simulink model "Citation_FlightGear_v2"  (R2026a)
settings: Solver=ode5  StopTime=40  FixedStep=0.01  EnableMultiTasking=on
InitFcn:
  | run('initcit.m')
  | run('id_init.m')
values from neighbouring files (symbols this model uses):
  cv1 = 20000    [gear_params.m]
  cv2 = cv1    (= 20000)    [gear_params.m]
  cv3 = 4000    [gear_params.m]
  cv4 = 20000    [gear_params.m]
  deltagmax1 = 0.25    [gear_params.m]
  deltagmax2 = deltagmax1    (= 0.25)    [gear_params.m]
  deltagmax3 = 0.24    [gear_params.m]
  deltagmax4 = 0.02    [gear_params.m]
  kt1 = 525020    [gear_params.m]
  kt2 = kt1    (= 525020)    [gear_params.m]
  kt3 = 457050    [gear_params.m]
  murol = 0.03*10    (= 0.3)    [gear_params.m]
  P1 = 2000    [gear_params.m]
  P2 = P1    (= 2000)    [gear_params.m]
  P3 = 2550    [gear_params.m]
  P4 = 40000    [gear_params.m]
  PL0 = 10000*eye(6)    [id_init.m]
  PM0 = 10000*eye(4)    [id_init.m]
  PN0 = 10000*eye(6)    [id_init.m]
  PX0 = 10000*eye(5)    [id_init.m]
  PY0 = 10000*eye(6)    [id_init.m]
  PZ0 = 10000*eye(4)    [id_init.m]
  thetaL0 = zeros(6,1)    [id_init.m]
  thetaM0 = zeros(4,1)    [id_init.m]
  thetaN0 = zeros(6,1)    [id_init.m]
  thetaX0 = zeros(5,1)    [id_init.m]
  thetaY0 = zeros(6,1)    [id_init.m]
  thetaZ0 = zeros(4,1)    [id_init.m]
  TL = 7.0875e-06    [id_init.m]    (also in plot_comparison_step_4.m = T_var(4))
  TM = 3.2564e-06    [id_init.m]    (also in plot_comparison_step_4.m = T_var(5))
  TN = 5.4692e-07    [id_init.m]    (also in plot_comparison_step_4.m = T_var(6))
  TX = 2.2784e-06    [id_init.m]    (also in plot_comparison_step_4.m = T_var(1))
  TY = 8.0633e-07    [id_init.m]    (also in plot_comparison_step_4.m = T_var(2))
  TZ = 2.8004e-05    [id_init.m]    (also in plot_comparison_step_4.m = T_var(3))
  xl1 = xcg-6.858    [gear_params.m]
  xl2 = xcg-6.858    [gear_params.m]
  xl3 = xcg-2.0752    [gear_params.m]
  xl4 = xcg-12.742    [gear_params.m]
  yl1 = 1.918    [gear_params.m]
  yl2 = -1.918    [gear_params.m]
  yl3 = 0    [gear_params.m]
  yl4 = 0    [gear_params.m]
  zl1 = zcg-1.701    [gear_params.m]
  zl2 = zcg-1.701    [gear_params.m]
  zl3 = zcg-1.7488    [gear_params.m]
  zl4 = zcg-2.78    [gear_params.m]
undefined symbols (not defined in the file or in its folder): chord, Deng, ealphag, ealphas, g0, hDME, hGS, lh, massinit, matbuaf, matdaf, matdam, matdbbf, matdeaf, matdgaf, matdqaf, matduaf, matdwaw, matedhr, mateif, matelhr, matemhr, matemv1, matemv2, matemve, matetam, mateuaf, matfaaf, matfaxl, matff, matibaf, matibb, matibmh, matipaf, matipmh, matiraf, matiuaf, matiwaf, matlaf, matlam, matleaf, matleam, matlgaf, matlqaf, matluaf, matmaaf, matmaam, matmaf, matmam, matmbbf, matmeaf, matmeam, matmgaf, matmqaf, matmrbr, matn1d, matn2d, matnbab, matnbaf, matnbmh ... (+53)
libraries: simulink x12, aerolibfltsims x3, aerolibconvert2 x2, aerolibobsolete x1, aerolibanimutils x1
(part 2 of 5)

== system Citation_FlightGear_v2/Cessna Citation 500/Citation model DASMAT/AIRCRAFT MODEL/EQM ==
  "FMtot " : Inport
  FMa : Inport  Port=2
  FMadot : Inport  Port=3
  FMbdot : Inport  Port=4
  massinit : Inport  Port=5
  wind : Inport  Port=6
  CFMa correction : Subsystem
  Integrator : Integrator  InitialCondition=x0
  State Derivatives : Subsystem
  x : Outport
  xdot : Outport  Port=2
  yuvw : Outport  Port=3
  FMtot corrected : Outport  Port=4
  FMa corrected : Outport  Port=5
  wires:
  State Derivatives/2(yuvw) -> yuvw/1
  State Derivatives/3(FMtot corrected) -> FMtot corrected/1
  FMa/1 -> CFMa correction/2(FMa)
  State Derivatives/1(xdot) -> xdot/1, CFMa correction/1(xdot), Integrator/1
  CFMa correction/1(FMa corrected) -> FMa corrected/1
  massinit/1 -> State Derivatives/5(massinit)
  "FMtot "/1 -> State Derivatives/2(FMtot)
  FMadot/1 -> CFMa correction/3(FMadot), State Derivatives/3(FMadot)
  FMbdot/1 -> CFMa correction/4(FMbdot), State Derivatives/4(FMbdot)
  Integrator/1 -> State Derivatives/1(x), x/1
  wind/1 -> State Derivatives/6(wind)

== system Citation_FlightGear_v2/Cessna Citation 500/Citation model DASMAT/AIRCRAFT MODEL/FM SORT ==
  FMa : Inport
  FMag : Inport  Port=2
  FMt : Inport  Port=3
  "Fgr " : Inport  Port=4
  Fgear : Inport  Port=5
  Mux : Mux  Inputs=[12 12]
  Sum : Sum  Inputs=+++++  InputSameDT=on  SaturateOnIntegerOverflow=on  OutDataTypeStr=Inherit: Same as first input
  Sum1 : Sum  Inputs=++++  InputSameDT=on  SaturateOnIntegerOverflow=on  OutDataTypeStr=Inherit: Same as first input
  aero : Demux  Outputs=[12 12]
      settings: DisplayOption=none
  engine : Demux  Outputs=[12 12]
      settings: DisplayOption=none
  gear : Demux  Outputs=[12 12]
      settings: DisplayOption=none
  gust : Demux  Outputs=[12 12]
      settings: DisplayOption=none
  FMtot : Outport
  wires:
  FMt/1 -> engine/1
  FMa/1 -> aero/1
  FMag/1 -> gust/1
  gust/2 -> Sum1/2
  Sum1/1 -> Mux/2
  engine/2 -> Sum1/3
  aero/2 -> Sum1/1
  gust/1 -> Sum/2
  engine/1 -> Sum/3
  Sum/1 -> Mux/1
  "Fgr "/1 -> Sum/4
  aero/1 -> Sum/1
  Mux/1 -> FMtot/1
  Fgear/1 -> gear/1
  gear/1 -> Sum/5
  gear/2 -> Sum1/4

== system Citation_FlightGear_v2/Cessna Citation 500/Citation model DASMAT/AIRCRAFT MODEL/GRAVITY ==
  "x " : Inport
  massinit : Inport  Port=2
  yatm : Inport  Port=3
  Fgr transformation : S-Function  FunctionName=ac_axes  Parameters=3  SFunctionDeploymentMode=off  EnableBusSupport=off
  Mux : Mux  Inputs=[12 3]
  Mux1 : Mux  Inputs=3
  Terminator_{1..9} (9 alike) : Terminator
  W : Product  InputSameDT=on  SaturateOnIntegerOverflow=on  OutDataTypeStr=Inherit: Same as first input
  atmosphere : Demux  Outputs=8
      settings: DisplayOption=none
  mass cg inertia : Demux  Outputs=[1 3 4]
      settings: DisplayOption=none
  zero : Constant  Value=0
  Fgr : Outport
  wires:
  mass cg inertia/3 -> Terminator_9/1
  mass cg inertia/2 -> Terminator_8/1
  atmosphere/8 -> Terminator_7/1
  atmosphere/7 -> Terminator_6/1
  atmosphere/6 -> Terminator_5/1
  atmosphere/5 -> Terminator_4/1
  atmosphere/3 -> Terminator_3/1
  atmosphere/2 -> Terminator_2/1
  atmosphere/1 -> Terminator_1/1
  Mux/1 -> Fgr transformation/1
  "x "/1 -> Mux/1
  Fgr transformation/1 -> Fgr/1
  mass cg inertia/1 -> W/1
  massinit/1 -> mass cg inertia/1
  yatm/1 -> atmosphere/1
  W/1 -> Mux1/3
  Mux1/1 -> Mux/2
  zero/1 -> Mux1/1, Mux1/2
  atmosphere/4 -> W/2

== system Citation_FlightGear_v2/Cessna Citation 500/Citation model DASMAT/AIRCRAFT MODEL/LANDING GEAR ==
  note: Landing Gear Model
      | Cessna Citation 500
      | Version 0.04NLR
      | (c) A.R. Veldhuijzen September 2001
  x : Inport
  xdot : Inport  Port=2
  massinit : Inport  Port=3
  ua : Inport  Port=4
  terr elev : Inport  Port=5
  Gear axes-cg transformation : Subsystem
  Landing Gear model : Subsystem
  Switch : Switch  Threshold=0.95  InputSameDT=off
  gear position : Selector  IndexOptions=Index vector (dialog)  Indices=[8]  OutputSizes=1
  zero : Constant  Value=[0 0 0 0 0 0]
  Fmt : Outport
  wires:
  xdot/1 -> Landing Gear model/2(xdot)
  x/1 -> Landing Gear model/1(x), Gear axes-cg transformation/2("x ")
  massinit/1 -> Gear axes-cg transformation/3(massinit)
  Gear axes-cg transformation/1(FMt) -> Fmt/1
  zero/1 -> Switch/1
  Landing Gear model/1(Forces and Moments) -> Switch/3
  Switch/1 -> Gear axes-cg transformation/1(FMt model)
  ua/1 -> gear position/1
  gear position/1 -> Switch/2
  terr elev/1 -> Landing Gear model/3(terrain elevation)

== system Citation_FlightGear_v2/Cessna Citation 500/Citation model DASMAT/AIRCRAFT MODEL/OBSERVATIONS ==
  note: Modified by Alex : Flight-Path Subsystem from Ac_mod instead of Ac_modpc
  x : Inport
  xdot : Inport  Port=2
  yuvw : Inport  Port=3
  FMtot : Inport  Port=4
  FMa : Inport  Port=5
  Fgr : Inport  Port=6
  massinit : Inport  Port=7
  yatm : Inport  Port=8
  Acceleration : Subsystem
  Energy : Subsystem
  Flight-Path : Subsystem
  yacc : Outport
  yfp : Outport  Port=2
  ys : Outport  Port=3
  wires:
  yuvw/1 -> Flight-Path/3(yuvw)
  Flight-Path/1(yfp) -> yfp/1
  Energy/1(ys) -> ys/1
  Acceleration/1(yacc) -> yacc/1
  FMa/1 -> Acceleration/4(FMa)
  Fgr/1 -> Acceleration/5(Fgr)
  yatm/1 -> Energy/3(yatm)
  FMtot/1 -> Acceleration/3(FMtot)
  Acceleration/2(acc earth) -> Flight-Path/4(acc earth)
  x/1 -> Flight-Path/1(x), Energy/1(x), Acceleration/1(x)
  xdot/1 -> Flight-Path/2(xdot), Energy/2(xdot), Acceleration/2(xdot)
  massinit/1 -> Acceleration/6(massinit)

== system Citation_FlightGear_v2/Cessna Citation 500/Citation model DASMAT/AIRCRAFT MODEL/WIND//TURBULENCE ==
  "x " : Inport
  Logarithmic Wind model : Subsystem
  Mux : Mux  Inputs=[12 3]
  Vwind transformation : S-Function  FunctionName=ac_axes  Parameters=3  SFunctionDeploymentMode=off  EnableBusSupport=off
  wind : Outport
  wires:
  Mux/1 -> Vwind transformation/1
  Vwind transformation/1 -> wind/1
  "x "/1 -> Mux/1, Logarithmic Wind model/1(In1)
  Logarithmic Wind model/1(Out1) -> Mux/2

== system Citation_FlightGear_v2/Pilot/Virtual Joystick (if you don't have a real one!)/Virtual Joystick/Throttle setting ==
  Demux : Demux  Tag=STV Demux  Outputs=1
      settings: DisplayOption=none
  FromWs : FromWorkspace  Tag=STV FromWs  VariableName=tuvar
      SigBuilderData=|
      | common.afterFinalStr = 'Extrapolate'
      | common.sampleTime = 0
      | dataSet.timeRange = [0 30]
      | dataSet.name = 'Group 1'
      | sbobj.Groups.Name = 'Group 1'
      | sbobj.Groups.Signals.Name = 'Signal 1'
      | sbobj.Groups.Signals.XData = [0 30]
      | sbobj.Groups.Signals.YData = [0.695 0.695]
      | sbobj.Groups.TimeRange = [0 30]
  Signal 1 : Outport  Tag=STV Outport
  wires:
  Demux/1 -> Signal 1/1
  FromWs/1 -> Demux/1

== system Citation_FlightGear_v2/Pilot/Virtual Joystick (if you don't have a real one!)/Virtual Joystick/delta aileron ==
  Demux : Demux  Tag=STV Demux  Outputs=3
      settings: DisplayOption=none
  FromWs : FromWorkspace  Tag=STV FromWs  VariableName=tuvar
      SigBuilderData=|
      | common.afterFinalStr = 'Extrapolate'
      | common.sampleTime = 0
      | dataSet.timeRange = [0 40]
      | dataSet.name = 'Group 1'
      | sbobj.Groups.Name = 'Group 1'
      | sbobj.Groups.Signals(1).Name = 'Signal 1'
      | sbobj.Groups.Signals(1).XData = [0 5 5 18 18 40]
      | sbobj.Groups.Signals(1).YData = [0 0 0.152 0.152 0 0]
      | sbobj.Groups.Signals(2).Name = 'Signal 2'
      | sbobj.Groups.Signals(2).XData = [0 25 25 28 28 40]
      | sbobj.Groups.Signals(2).YData = [0 0 -0.07 -0.07 0 0]
      | sbobj.Groups.Signals(3).Name = 'Signal 3'
      | sbobj.Groups.Signals(3).XData = [0 28 28 40]
      | sbobj.Groups.Signals(3).YData = [0 0 -0.04 -0.04]
      | sbobj.Groups.TimeRange = [0 40]
  Signal 1 : Outport  Tag=STV Outport
  Signal 2 : Outport  Tag=STV Outport  Port=2
  Signal 3 : Outport  Tag=STV Outport  Port=3
  wires:
  Demux/1 -> Signal 1/1
  FromWs/1 -> Demux/1
  Demux/2 -> Signal 2/1
  Demux/3 -> Signal 3/1

== system Citation_FlightGear_v2/Pilot/Virtual Joystick (if you don't have a real one!)/Virtual Joystick/delta elevator ==
  Demux : Demux  Tag=STV Demux  Outputs=1
      settings: DisplayOption=none
  FromWs : FromWorkspace  Tag=STV FromWs  VariableName=tuvar
      SigBuilderData=|
      | common.afterFinalStr = 'Extrapolate'
      | common.sampleTime = 0
      | dataSet.timeRange = [0 100]
      | dataSet.name = 'Group 1'
      | sbobj.Groups.Name = 'Group 1'
      | sbobj.Groups.Signals.Name = 'Signal 1'
      | sbobj.Groups.Signals.XData = [0 5 100]
      | sbobj.Groups.Signals.YData = [-0.02795 -0.02795 -0.02795]
      | sbobj.Groups.TimeRange = [0 100]
  Signal 1 : Outport  Tag=STV Outport
  wires:
  Demux/1 -> Signal 1/1
  FromWs/1 -> Demux/1

== system Citation_FlightGear_v2/Pilot/Virtual Joystick (if you don't have a real one!)/Virtual Joystick/delta rudder ==
  Demux : Demux  Tag=STV Demux  Outputs=1
      settings: DisplayOption=none
  FromWs : FromWorkspace  Tag=STV FromWs  VariableName=tuvar
      SigBuilderData=|
      | common.afterFinalStr = 'Extrapolate'
      | common.sampleTime = 0
      | dataSet.timeRange = [0 30]
      | dataSet.name = 'Group 1'
      | sbobj.Groups.Name = 'Group 1'
      | sbobj.Groups.Signals.Name = 'Signal 1'
      | sbobj.Groups.Signals.XData = [0 4 6 30]
      | sbobj.Groups.Signals.YData = [0 0 0 0]
      | sbobj.Groups.TimeRange = [0 30]
  Signal 1 : Outport  Tag=STV Outport
  wires:
  Demux/1 -> Signal 1/1
  FromWs/1 -> Demux/1

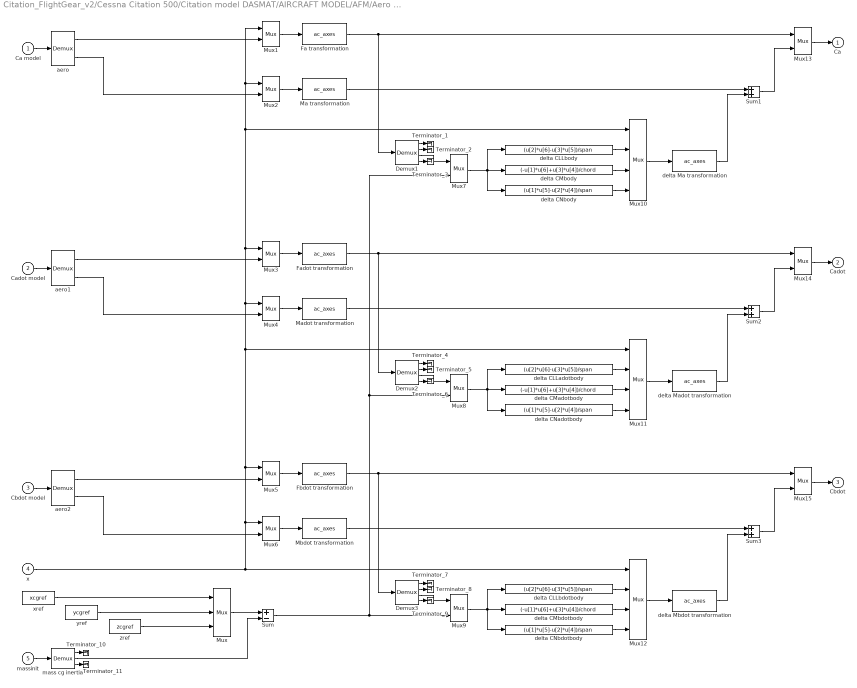
== system Citation_FlightGear_v2/Cessna Citation 500/Citation model DASMAT/AIRCRAFT MODEL/AFM/Aero axes-cg transformation ==
  Ca model : Inport
  Cadot model : Inport  Port=2
  Cbdot model : Inport  Port=3
  "x " : Inport  Port=4
  massinit : Inport  Port=5
  Demux1 : Demux  Outputs=[3 3 3 3]
      settings: DisplayOption=none
  Demux2 : Demux  Outputs=[3 3 3 3]
      settings: DisplayOption=none
  Demux3 : Demux  Outputs=[3 3 3 3]
      settings: DisplayOption=none
  Fa transformation : S-Function  FunctionName=ac_axes  Parameters=axes_CFMaero  SFunctionDeploymentMode=off  EnableBusSupport=off
  Fadot transformation : S-Function  FunctionName=ac_axes  Parameters=axes_CFMaero  SFunctionDeploymentMode=off  EnableBusSupport=off
  Fbdot transformation : S-Function  FunctionName=ac_axes  Parameters=axes_CFMaero  SFunctionDeploymentMode=off  EnableBusSupport=off
  Ma transformation : S-Function  FunctionName=ac_axes  Parameters=axes_CFMaero  SFunctionDeploymentMode=off  EnableBusSupport=off
  Madot transformation : S-Function  FunctionName=ac_axes  Parameters=axes_CFMaero  SFunctionDeploymentMode=off  EnableBusSupport=off
  Mbdot transformation : S-Function  FunctionName=ac_axes  Parameters=axes_CFMaero  SFunctionDeploymentMode=off  EnableBusSupport=off
  Mux : Mux  Inputs=3
  Mux{1..6} (6 alike) : Mux  Inputs=[12 3]
  Mux10 : Mux  Inputs=[12 1 1 1]
  Mux11 : Mux  Inputs=[12 1 1 1]
  Mux12 : Mux  Inputs=[12 1 1 1]
  Mux13 : Mux  Inputs=[12 12]
  Mux14 : Mux  Inputs=[12 12]
  Mux15 : Mux  Inputs=[12 12]
  Mux7 : Mux  Inputs=[3 3]
  Mux8 : Mux  Inputs=[3 3]
  Mux9 : Mux  Inputs=[3 3]
  Sum : Sum  Inputs=+-  InputSameDT=on  SaturateOnIntegerOverflow=on  OutDataTypeStr=Inherit: Same as first input
  Sum1 : Sum  InputSameDT=on  SaturateOnIntegerOverflow=on  OutDataTypeStr=Inherit: Same as first input
  Sum2 : Sum  InputSameDT=on  SaturateOnIntegerOverflow=on  OutDataTypeStr=Inherit: Same as first input
  Sum3 : Sum  InputSameDT=on  SaturateOnIntegerOverflow=on  OutDataTypeStr=Inherit: Same as first input
  Terminator_{1..11} (11 alike) : Terminator
  aero : Demux  Outputs=[3 3]
      settings: DisplayOption=none
  aero1 : Demux  Outputs=[3 3]
      settings: DisplayOption=none
  aero2 : Demux  Outputs=[3 3]
      settings: DisplayOption=none
  delta CLLadotbody : Fcn  Expr=(u[2]*u[6]-u[3]*u[5])/span
  delta CLLbdotbody : Fcn  Expr=(u[2]*u[6]-u[3]*u[5])/span
  delta CLLbody : Fcn  Expr=(u[2]*u[6]-u[3]*u[5])/span
  delta CMadotbody : Fcn  Expr=(-u[1]*u[6]+u[3]*u[4])/chord
  delta CMbdotbody : Fcn  Expr=(-u[1]*u[6]+u[3]*u[4])/chord
  delta CMbody : Fcn  Expr=(-u[1]*u[6]+u[3]*u[4])/chord
  delta CNadotbody : Fcn  Expr=(u[1]*u[5]-u[2]*u[4])/span
  delta CNbdotbody : Fcn  Expr=(u[1]*u[5]-u[2]*u[4])/span
  delta CNbody : Fcn  Expr=(u[1]*u[5]-u[2]*u[4])/span
  delta Ma transformation : S-Function  FunctionName=ac_axes  Parameters=2  SFunctionDeploymentMode=off  EnableBusSupport=off
  delta Madot transformation : S-Function  FunctionName=ac_axes  Parameters=2  SFunctionDeploymentMode=off  EnableBusSupport=off
  delta Mbdot transformation : S-Function  FunctionName=ac_axes  Parameters=2  SFunctionDeploymentMode=off  EnableBusSupport=off
  mass cg inertia : Demux  Outputs=[1 3 4]
      settings: DisplayOption=none
  xref : Constant  Value=xcgref
  yref : Constant  Value=ycgref
  zref : Constant  Value=zcgref
  Ca : Outport
  Cadot : Outport  Port=2
  Cbdot : Outport  Port=3
  wires:
  mass cg inertia/3 -> Terminator_11/1
  mass cg inertia/1 -> Terminator_10/1
  Demux3/4 -> Terminator_9/1
  Demux3/2 -> Terminator_8/1
  Demux3/1 -> Terminator_7/1
  Demux2/4 -> Terminator_6/1
  Demux2/2 -> Terminator_5/1
  Demux2/1 -> Terminator_4/1
  Demux1/4 -> Terminator_3/1
  Demux1/2 -> Terminator_2/1
  Demux1/1 -> Terminator_1/1
  aero1/1 -> Mux3/2
  Cadot model/1 -> aero1/1
  aero1/2 -> Mux4/2
  Ca model/1 -> aero/1
  massinit/1 -> mass cg inertia/1
  aero/1 -> Mux1/2
  xref/1 -> Mux/1
  yref/1 -> Mux/2
  zref/1 -> Mux/3
  mass cg inertia/2 -> Sum/2
  Mux/1 -> Sum/1
  Fa transformation/1 -> Demux1/1, Mux13/1
  Mux7/1 -> delta CLLbody/1, delta CNbody/1, delta CMbody/1
  delta CLLbody/1 -> Mux10/2
  delta CMbody/1 -> Mux10/3
  delta CNbody/1 -> Mux10/4
  Mux10/1 -> delta Ma transformation/1
  Ma transformation/1 -> Sum1/1
  Sum1/1 -> Mux13/2
  Mux13/1 -> Ca/1
  Mux1/1 -> Fa transformation/1
  Mux3/1 -> Fadot transformation/1
  Mux14/1 -> Cadot/1
  Sum2/1 -> Mux14/2
  Madot transformation/1 -> Sum2/1
  Mux12/1 -> delta Mbdot transformation/1
  delta CNbdotbody/1 -> Mux12/4
  delta CMbdotbody/1 -> Mux12/3
  delta CLLbdotbody/1 -> Mux12/2
  Mux9/1 -> delta CLLbdotbody/1, delta CNbdotbody/1, delta CMbdotbody/1
  Mux4/1 -> Madot transformation/1
  Mux2/1 -> Ma transformation/1
  aero/2 -> Mux2/2
  delta Ma transformation/1 -> Sum1/2
  Demux1/3 -> Mux7/1
  Demux3/3 -> Mux9/1
  Demux2/3 -> Mux8/1
  Mux11/1 -> delta Madot transformation/1
  delta CNadotbody/1 -> Mux11/4
  delta CMadotbody/1 -> Mux11/3
  delta CLLadotbody/1 -> Mux11/2
  Mux8/1 -> delta CLLadotbody/1, delta CNadotbody/1, delta CMadotbody/1
  Fadot transformation/1 -> Demux2/1, Mux14/1
  delta Madot transformation/1 -> Sum2/2
  Sum/1 -> Mux8/2, Mux7/2, Mux9/2
  Mux6/1 -> Mbdot transformation/1
  Mux5/1 -> Fbdot transformation/1
  aero2/2 -> Mux6/2
  Cbdot model/1 -> aero2/1
  aero2/1 -> Mux5/2
  "x "/1 -> Mux4/1, Mux3/1, Mux2/1, Mux1/1, Mux10/1, Mux11/1, Mux5/1, Mux6/1, Mux12/1
  Mbdot transformation/1 -> Sum3/1
  Fbdot transformation/1 -> Demux3/1, Mux15/1
  Sum3/1 -> Mux15/2
  delta Mbdot transformation/1 -> Sum3/2
  Mux15/1 -> Cbdot/1

== system Citation_FlightGear_v2/Cessna Citation 500/Citation model DASMAT/AIRCRAFT MODEL/AFM/Aeromod ==
  x : Inport
  ua : Inport  Port=2
  massinit : Inport  Port=3
  yad1 : Inport  Port=4
  yad2 : Inport  Port=5
  gust : Inport  Port=6
  yatm : Inport  Port=7
  Demux : Demux  Outputs=[6 6 6 6]
      settings: DisplayOption=none
  Mux1 : Mux  Inputs=24
  SubSystem : Subsystem
  cg selector : Selector  IndexOptions=Index vector (dialog)  Indices=[2 3 4]  OutputSizes=1
  Ca : Outport
  Cadot : Outport  Port=2
  Cbdot : Outport  Port=3
  Cag : Outport  Port=4
  wires:
  Mux1/1 -> Demux/1
  Demux/1 -> Ca/1
  Demux/2 -> Cadot/1
  Demux/3 -> Cbdot/1
  Demux/4 -> Cag/1
  SubSystem/2(CY) -> Mux1/2
  SubSystem/3(CZ) -> Mux1/3
  SubSystem/5(CM) -> Mux1/5
  SubSystem/6(CN) -> Mux1/6
  SubSystem/8(CYadot) -> Mux1/8
  SubSystem/9(CZadot) -> Mux1/9
  SubSystem/11(CMadot) -> Mux1/11
  SubSystem/12(CNadot) -> Mux1/12
  SubSystem/14(CYbdot) -> Mux1/14
  SubSystem/15(CZbdot) -> Mux1/15
  SubSystem/17(CMbdot) -> Mux1/17
  SubSystem/18(CNbdot) -> Mux1/18
  SubSystem/20(CYg) -> Mux1/20
  SubSystem/21(CZg) -> Mux1/21
  SubSystem/23(CMg) -> Mux1/23
  SubSystem/24(CNg) -> Mux1/24
  SubSystem/22(CLLg) -> Mux1/22
  SubSystem/19(CXg) -> Mux1/19
  SubSystem/16(CLLbdot) -> Mux1/16
  SubSystem/13(CXbdot) -> Mux1/13
  SubSystem/10(CLLadot) -> Mux1/10
  SubSystem/7(CXadot) -> Mux1/7
  SubSystem/4(CLL) -> Mux1/4
  SubSystem/1(CX) -> Mux1/1
  massinit/1 -> cg selector/1
  yad1/1 -> SubSystem/4(yad1)
  gust/1 -> SubSystem/6(gust)
  yad2/1 -> SubSystem/5(yad2)
  ua/1 -> SubSystem/2(ua)
  x/1 -> SubSystem/1(x)
  cg selector/1 -> SubSystem/3(cg)
  yatm/1 -> SubSystem/7(yatm)

== system Citation_FlightGear_v2/Cessna Citation 500/Citation model DASMAT/AIRCRAFT MODEL/AFM/FMaerodims ==
  Ca : Inport
  Cadot : Inport  Port=2
  Cbdot : Inport  Port=3
  x : Inport  Port=4
  yad1 : Inport  Port=5
  Prod : Product  InputSameDT=on  SaturateOnIntegerOverflow=on  OutDataTypeStr=Inherit: Same as first input
  Prod1 : Product  Inputs=3  InputSameDT=on  SaturateOnIntegerOverflow=on  OutDataTypeStr=Inherit: Same as first input
  Prod2 : Product  Inputs=3  InputSameDT=on  SaturateOnIntegerOverflow=on  OutDataTypeStr=Inherit: Same as first input
  b/V : Fcn  Expr=span/u[4]
  c/V : Fcn  Expr=chord/u[4]
  dims : Subsystem
  dims1 : Subsystem
  dims2 : Subsystem
  qdyn*S : Fcn  Expr=u[2]*S
  FMa : Outport
  FMadot : Outport  Port=2
  FMbdot : Outport  Port=3
  wires:
  Ca/1 -> Prod/1
  Prod/1 -> dims/1(FM/length)
  dims/1(FM) -> FMa/1
  yad1/1 -> qdyn*S/1
  Cbdot/1 -> Prod2/1
  qdyn*S/1 -> Prod2/2, Prod1/2, Prod/2
  Cadot/1 -> Prod1/1
  Prod1/1 -> dims1/1(F FM/length)
  dims1/1(FM) -> FMadot/1
  Prod2/1 -> dims2/1(F FM/length)
  dims2/1(FM) -> FMbdot/1
  x/1 -> b/V/1, c/V/1
  c/V/1 -> Prod1/3
  b/V/1 -> Prod2/3

== system Citation_FlightGear_v2/Cessna Citation 500/Citation model DASMAT/AIRCRAFT MODEL/AFM/FMgustdims ==
  Cag : Inport
  yad1 : Inport  Port=2
  Prod : Product  InputSameDT=on  SaturateOnIntegerOverflow=on  OutDataTypeStr=Inherit: Same as first input
  dims : Subsystem
  qdyn*S : Fcn  Expr=u[2]*S
  FMag : Outport
  wires:
  Cag/1 -> Prod/1
  Prod/1 -> dims/1(F M/length)
  yad1/1 -> qdyn*S/1
  dims/1(FM) -> FMag/1
  qdyn*S/1 -> Prod/2

== system Citation_FlightGear_v2/Cessna Citation 500/Citation model DASMAT/AIRCRAFT MODEL/AFM/Gust axes-cg transformation ==
  Cag model : Inport
  "x " : Inport  Port=2
  massinit : Inport  Port=3
  Demux1 : Demux  Outputs=[3 3 3 3]
      settings: DisplayOption=none
  Fag transformation : S-Function  FunctionName=ac_axes  Parameters=axes_CFMgust  SFunctionDeploymentMode=off  EnableBusSupport=off
  Mag transformation : S-Function  FunctionName=ac_axes  Parameters=axes_CFMgust  SFunctionDeploymentMode=off  EnableBusSupport=off
  Mux1 : Mux  Inputs=[12 3]
  Mux2 : Mux  Inputs=[12 3]
  Mux3 : Mux  Inputs=[3 3]
  Mux4 : Mux  Inputs=[12 1 1 1]
  Mux5 : Mux  Inputs=[12 12]
  Mux6 : Mux  Inputs=3
  Sum : Sum  Inputs=+-  InputSameDT=on  SaturateOnIntegerOverflow=on  OutDataTypeStr=Inherit: Same as first input
  Sum1 : Sum  InputSameDT=on  SaturateOnIntegerOverflow=on  OutDataTypeStr=Inherit: Same as first input
  Terminator_{1..5} (5 alike) : Terminator
  delta CLLbody : Fcn  Expr=(u[2]*u[6]-u[3]*u[5])/span
  delta CMbody : Fcn  Expr=(-u[1]*u[6]+u[3]*u[4])/chord
  delta CNbody : Fcn  Expr=(u[1]*u[5]-u[2]*u[4])/span
  delta Mag transformation : S-Function  FunctionName=ac_axes  Parameters=2  SFunctionDeploymentMode=off  EnableBusSupport=off
  gust : Demux  Outputs=[3 3]
      settings: DisplayOption=none
  mass cg inertia : Demux  Outputs=[1 3 4]
      settings: DisplayOption=none
  xref : Constant  Value=xcgref
  yref : Constant  Value=ycgref
  zref : Constant  Value=zcgref
  Cag : Outport
  wires:
  mass cg inertia/3 -> Terminator_5/1
  mass cg inertia/1 -> Terminator_4/1
  Demux1/4 -> Terminator_3/1
  Demux1/2 -> Terminator_2/1
  Demux1/1 -> Terminator_1/1
  Cag model/1 -> gust/1
  massinit/1 -> mass cg inertia/1
  gust/1 -> Mux1/2
  xref/1 -> Mux6/1
  yref/1 -> Mux6/2
  zref/1 -> Mux6/3
  mass cg inertia/2 -> Sum/2
  Mux6/1 -> Sum/1
  Fag transformation/1 -> Demux1/1, Mux5/1
  Mag transformation/1 -> Sum1/1
  Sum1/1 -> Mux5/2
  Mux5/1 -> Cag/1
  Mux1/1 -> Fag transformation/1
  delta Mag transformation/1 -> Sum1/2
  Mux2/1 -> Mag transformation/1
  Sum/1 -> Mux3/2
  gust/2 -> Mux2/2
  "x "/1 -> Mux2/1, Mux1/1, Mux4/1
  Mux3/1 -> delta CLLbody/1, delta CNbody/1, delta CMbody/1
  delta CLLbody/1 -> Mux4/2
  delta CMbody/1 -> Mux4/3
  delta CNbody/1 -> Mux4/4
  Demux1/3 -> Mux3/1
  Mux4/1 -> delta Mag transformation/1

== system Citation_FlightGear_v2/Cessna Citation 500/Citation model DASMAT/AIRCRAFT MODEL/EFM/Engine axes-cg transformation ==
  FMt model : Inport
  "x " : Inport  Port=2
  massinit : Inport  Port=3
  Demux : Demux  Outputs=[3 3 3 3]
      settings: DisplayOption=none
  Ft transformation : S-Function  FunctionName=ac_axes  Parameters=2  SFunctionDeploymentMode=off  EnableBusSupport=off
  Mt transformation : S-Function  FunctionName=ac_axes  Parameters=2  SFunctionDeploymentMode=off  EnableBusSupport=off
  Mux1 : Mux  Inputs=[12 3]
  Mux2 : Mux  Inputs=[12 3]
  Mux3 : Mux  Inputs=[3 3]
  Mux4 : Mux  Inputs=[12 1 1 1]
  Mux5 : Mux  Inputs=[12 12]
  "Neg " : Gain  Gain=-1  SaturateOnIntegerOverflow=on  OutDataTypeStr=Inherit: Same as input  ParamDataTypeStr=Inherit: Same as input
  Sum1 : Sum  InputSameDT=on  SaturateOnIntegerOverflow=on  OutDataTypeStr=Inherit: Same as first input
  Terminator_{1..5} (5 alike) : Terminator
  delta LLbody : Fcn  Expr=u[2]*u[6]-u[3]*u[5]
  delta Mbody : Fcn  Expr=-u[1]*u[6]+u[3]*u[4]
  delta Mt transformation : S-Function  FunctionName=ac_axes  Parameters=2  SFunctionDeploymentMode=off  EnableBusSupport=off
  delta Nbody : Fcn  Expr=u[1]*u[5]-u[2]*u[4]
  engine : Demux  Outputs=[3 3]
      settings: DisplayOption=none
  mass cg inertia : Demux  Outputs=[1 3 4]
      settings: DisplayOption=none
  FMt : Outport
  wires:
  mass cg inertia/3 -> Terminator_5/1
  mass cg inertia/1 -> Terminator_4/1
  Demux/4 -> Terminator_3/1
  Demux/2 -> Terminator_2/1
  Demux/1 -> Terminator_1/1
  FMt model/1 -> engine/1
  massinit/1 -> mass cg inertia/1
  engine/1 -> Mux1/2
  Ft transformation/1 -> Demux/1, Mux5/1
  Mt transformation/1 -> Sum1/1
  Sum1/1 -> Mux5/2
  Mux5/1 -> FMt/1
  Mux1/1 -> Ft transformation/1
  delta Mt transformation/1 -> Sum1/2
  Mux2/1 -> Mt transformation/1
  engine/2 -> Mux2/2
  "x "/1 -> Mux2/1, Mux1/1, Mux4/1
  Mux3/1 -> delta LLbody/1, delta Nbody/1, delta Mbody/1
  delta LLbody/1 -> Mux4/2
  delta Mbody/1 -> Mux4/3
  delta Nbody/1 -> Mux4/4
  Mux4/1 -> delta Mt transformation/1
  Demux/3 -> Mux3/1
  mass cg inertia/2 -> "Neg "/1
  "Neg "/1 -> Mux3/2

== system Citation_FlightGear_v2/Cessna Citation 500/Citation model DASMAT/AIRCRAFT MODEL/EFM/Engmod ==
  x : Inport
  ut : Inport  Port=2
  yatm : Inport  Port=3
  yad1 : Inport  Port=4
  yad2 : Inport  Port=5
  Citation eng_mod : Subsystem
  Mux : Mux  Inputs=[12 2 8 2 8]
  FMt : Outport
  ypp : Outport  Port=2
  wires:
  x/1 -> Mux/1
  ut/1 -> Mux/2
  yatm/1 -> Mux/3
  yad1/1 -> Mux/4
  yad2/1 -> Mux/5
  Mux/1 -> Citation eng_mod/1(In1)
  Citation eng_mod/1(Out1) -> FMt/1
  Citation eng_mod/2(ypp) -> ypp/1

== system Citation_FlightGear_v2/Cessna Citation 500/Citation model DASMAT/AIRCRAFT MODEL/EQM/CFMa correction ==
  xdot : Inport
  FMa : Inport  Port=2
  FMadot : Inport  Port=3
  FMbdot : Inport  Port=4
  Prod2 : Product  InputSameDT=on  SaturateOnIntegerOverflow=on  OutDataTypeStr=Inherit: Same as first input
  Prod3 : Product  InputSameDT=on  SaturateOnIntegerOverflow=on  OutDataTypeStr=Inherit: Same as first input
  Sum1 : Sum  Inputs=+++  InputSameDT=on  SaturateOnIntegerOverflow=on  OutDataTypeStr=Inherit: Same as first input
  Terminator_{1..10} (10 alike) : Terminator
  derivatives : Demux  Outputs=12
      settings: DisplayOption=none
  FMa corrected : Outport
  wires:
  derivatives/12 -> Terminator_10/1
  derivatives/11 -> Terminator_9/1
  derivatives/10 -> Terminator_8/1
  derivatives/9 -> Terminator_7/1
  derivatives/8 -> Terminator_6/1
  derivatives/7 -> Terminator_5/1
  derivatives/4 -> Terminator_4/1
  derivatives/3 -> Terminator_3/1
  derivatives/2 -> Terminator_2/1
  derivatives/1 -> Terminator_1/1
  xdot/1 -> derivatives/1
  Sum1/1 -> FMa corrected/1
  FMa/1 -> Sum1/1
  FMbdot/1 -> Prod3/1
  FMadot/1 -> Prod2/1
  Prod2/1 -> Sum1/2
  Prod3/1 -> Sum1/3
  derivatives/5 -> Prod2/2
  derivatives/6 -> Prod3/2

== system Citation_FlightGear_v2/Cessna Citation 500/Citation model DASMAT/AIRCRAFT MODEL/EQM/State Derivatives ==
  note: mass
  note: inertia
  x : Inport
  FMtot : Inport  Port=2
  FMadot : Inport  Port=3
  FMbdot : Inport  Port=4
  massinit : Inport  Port=5
  wind : Inport  Port=6
  Mux1 : Mux  Inputs=[12 12]
  Mux2 : Mux  Inputs=[3 3 3 3]
  Terminator_1 : Terminator
  Vabdot : Subsystem
  aero1 : Demux  Outputs=[12 12]
      settings: DisplayOption=none
  aero2 : Demux  Outputs=[12 12]
      settings: DisplayOption=none
  eulerdot : Subsystem
  hxydot : Subsystem
  mass properties : Subsystem
  pqrdot : Subsystem
  states transformation : Subsystem
  total : Demux  Outputs=[12 12]
      settings: DisplayOption=none
  xdot : Outport
  yuvw : Outport  Port=2
  FMtot corrected : Outport  Port=3
  wires:
  states transformation/3(ydl) -> Terminator_1/1
  wind/1 -> hxydot/2(wind), Vabdot/7(wind)
  total/1 -> Vabdot/3(Ftot)
  states transformation/2(yuvw) -> hxydot/1(yuvw), yuvw/1
  Mux1/1 -> FMtot corrected/1
  hxydot/1(hxydot) -> Mux2/4
  eulerdot/1(eulerdot) -> Mux2/3
  pqrdot/2(Mtot corrected) -> Mux1/2
  pqrdot/1(pqrdot) -> Mux2/1
  Vabdot/2(Ftot corrected) -> Mux1/1
  aero2/1 -> Vabdot/5(Fbdot)
  total/2 -> pqrdot/2(Mtot)
  mass properties/2(inertia) -> pqrdot/5(inertia)
  mass properties/1(mass) -> Vabdot/6(mass)
  aero1/1 -> Vabdot/4(Fadot)
  states transformation/1(ypqr) -> pqrdot/1(ypqr), Vabdot/2(ypqr)
  x/1 -> Vabdot/1(x), eulerdot/1(x), states transformation/1(x)
  aero2/2 -> pqrdot/4(Mbdot)
  aero1/2 -> pqrdot/3(Madot)
  Vabdot/1(Vabdot) -> pqrdot/6(Vabdot), Mux2/2
  FMbdot/1 -> aero2/1
  FMadot/1 -> aero1/1
  FMtot/1 -> total/1
  massinit/1 -> mass properties/1(massinit)
  Mux2/1 -> xdot/1

== system Citation_FlightGear_v2/Cessna Citation 500/Citation model DASMAT/AIRCRAFT MODEL/LANDING GEAR/Gear axes-cg transformation ==
  FMt model : Inport
  "x " : Inport  Port=2
  massinit : Inport  Port=3
  Demux : Demux  Outputs=[3 3 3 3]
      settings: DisplayOption=none
  Ft transformation : S-Function  FunctionName=ac_axes  Parameters=2  SFunctionDeploymentMode=off  EnableBusSupport=off
  Gear Forces and Moments : Demux  Outputs=[3 3]
      settings: DisplayOption=none
  Mt transformation : S-Function  FunctionName=ac_axes  Parameters=2  SFunctionDeploymentMode=off  EnableBusSupport=off
  Mux1 : Mux  Inputs=[12 3]
  Mux2 : Mux  Inputs=[12 3]
  Mux3 : Mux  Inputs=[3 3]
  Mux4 : Mux  Inputs=[12 1 1 1]
  Mux5 : Mux  Inputs=[12 12]
  "Neg " : Gain  Gain=-1  SaturateOnIntegerOverflow=on  OutDataTypeStr=Inherit: Same as input  ParamDataTypeStr=Inherit: Same as input
  Scope3 : Scope
  Scope4 : Scope
  Terminator_{1..6} (6 alike) : Terminator
  delta LLbody : Fcn  Expr=u[2]*u[6]-u[3]*u[5]
  delta Mbody : Fcn  Expr=-u[1]*u[6]+u[3]*u[4]
  delta Mt transformation : S-Function  FunctionName=ac_axes  Parameters=2  SFunctionDeploymentMode=off  EnableBusSupport=off
  delta Nbody : Fcn  Expr=u[1]*u[5]-u[2]*u[4]
  mass cg inertia : Demux  Outputs=[1 3 4]
      settings: DisplayOption=none
  FMt : Outport
  wires:
  mass cg inertia/3 -> Terminator_5/1
  mass cg inertia/1 -> Terminator_4/1
  Demux/4 -> Terminator_3/1
  Demux/2 -> Terminator_2/1
  Demux/1 -> Terminator_1/1
  FMt model/1 -> Gear Forces and Moments/1
  massinit/1 -> mass cg inertia/1
  Gear Forces and Moments/1 -> Mux1/2
  Ft transformation/1 -> Demux/1, Mux5/1
  Mux5/1 -> FMt/1
  Mux1/1 -> Ft transformation/1
  Mux2/1 -> Mt transformation/1
  Gear Forces and Moments/2 -> Mux2/2
  "x "/1 -> Mux2/1, Mux1/1, Mux4/1
  Mux3/1 -> delta LLbody/1, delta Nbody/1, delta Mbody/1
  delta LLbody/1 -> Mux4/2
  delta Mbody/1 -> Mux4/3
  delta Nbody/1 -> Mux4/4
  Mux4/1 -> delta Mt transformation/1
  Demux/3 -> Mux3/1
  mass cg inertia/2 -> "Neg "/1
  "Neg "/1 -> Mux3/2
  Mt transformation/1 -> Scope3/1, Mux5/2, Scope4/1
  delta Mt transformation/1 -> Terminator_6/1

== system Citation_FlightGear_v2/Cessna Citation 500/Citation model DASMAT/AIRCRAFT MODEL/LANDING GEAR/Landing Gear model ==
  note: NLR Model
  x : Inport
  xdot : Inport  Port=2
  terrain elevation : Inport  Port=3
  Correct for terrain elevation : Subsystem
  Left Main Gear : Subsystem
  Mux : Mux  Inputs=2
  Mux1 : Mux  Inputs=2
  Nose Gear : Subsystem
  Right Main Gear : Subsystem
  Sum : Sum  Inputs=++++  InputSameDT=on  SaturateOnIntegerOverflow=on  OutDataTypeStr=Inherit: Same as first input
  Sum1 : Sum  Inputs=++++  InputSameDT=on  SaturateOnIntegerOverflow=on  OutDataTypeStr=Inherit: Same as first input
  Tail Scraper : Subsystem
  hdot selector : Selector  IndexOptions=Index vector (dialog)  Indices=[10]  OutputSizes=1
  Forces and Moments : Outport
  wires:
  xdot/1 -> hdot selector/1
  Mux/1 -> Left Main Gear/1(Inputs), Nose Gear/1(Inputs), Right Main Gear/1(Inputs), Tail Scraper/1(Inputs)
  Mux1/1 -> Forces and Moments/1
  Correct for terrain elevation/1(x corrected) -> Mux/1
  x/1 -> Correct for terrain elevation/1(x)
  Tail Scraper/1(FX FY FZ) -> Sum/4
  Tail Scraper/2(L M N) -> Sum1/4
  Right Main Gear/1(FX FY FZ) -> Sum/3
  Nose Gear/2(L M N) -> Sum1/2
  Sum1/1 -> Mux1/2
  Sum/1 -> Mux1/1
  Left Main Gear/1(FX FY FZ) -> Sum/1
  Left Main Gear/2(L M N) -> Sum1/1
  Nose Gear/1(FX FY FZ) -> Sum/2
  Right Main Gear/2(L M N) -> Sum1/3
  terrain elevation/1 -> Correct for terrain elevation/2(terr elev)
  hdot selector/1 -> Mux/2

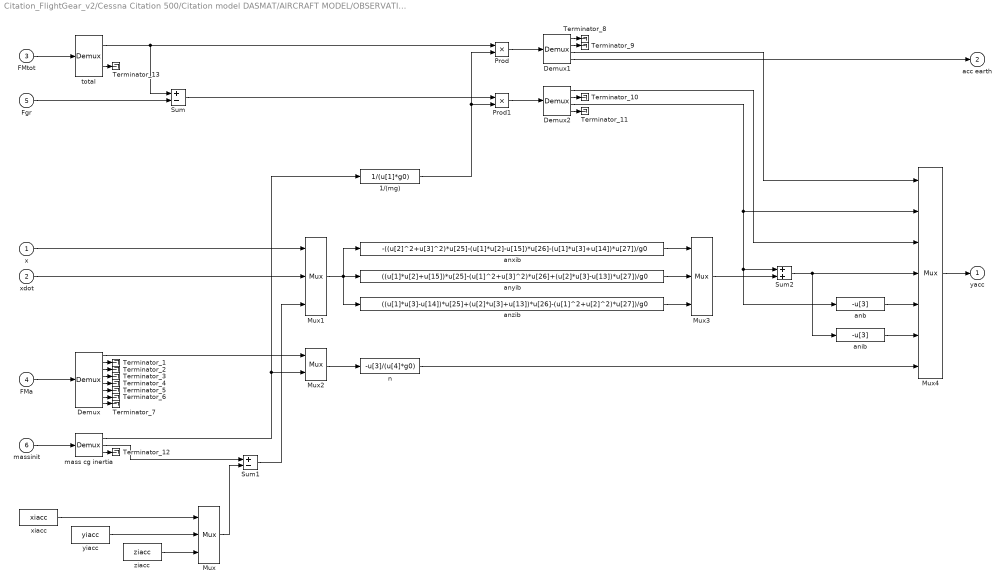
== system Citation_FlightGear_v2/Cessna Citation 500/Citation model DASMAT/AIRCRAFT MODEL/OBSERVATIONS/Acceleration ==
  x : Inport
  xdot : Inport  Port=2
  FMtot : Inport  Port=3
  FMa : Inport  Port=4
  Fgr : Inport  Port=5
  massinit : Inport  Port=6
  1/(mg) : Fcn  Expr=1/(u[1]*g0)
  Demux : Demux  Outputs=[3 3 3 3 3 3 3 3]
      settings: DisplayOption=none
  Demux1 : Demux  Outputs=[3 3 3 3]
      settings: DisplayOption=none
  Demux2 : Demux  Outputs=[3 3 3 3]
      settings: DisplayOption=none
  Mux : Mux  Inputs=3
  Mux1 : Mux  Inputs=[12 12 3]
  Mux2 : Mux  Inputs=[3 1]
  Mux3 : Mux  Inputs=3
  Mux4 : Mux  Inputs=[3 3 3 3 1 1 1]
  Prod : Product  InputSameDT=on  SaturateOnIntegerOverflow=on  OutDataTypeStr=Inherit: Same as first input
  Prod1 : Product  InputSameDT=on  SaturateOnIntegerOverflow=on  OutDataTypeStr=Inherit: Same as first input
  Sum : Sum  Inputs=+-  InputSameDT=on  SaturateOnIntegerOverflow=on  OutDataTypeStr=Inherit: Same as first input
  Sum1 : Sum  Inputs=+-  InputSameDT=on  SaturateOnIntegerOverflow=on  OutDataTypeStr=Inherit: Same as first input
  Sum2 : Sum  InputSameDT=on  SaturateOnIntegerOverflow=on  OutDataTypeStr=Inherit: Same as first input
  Terminator_{1..13} (13 alike) : Terminator
  anb : Fcn  Expr=-u[3]
  anib : Fcn  Expr=-u[3]
  anxib : Fcn  Expr=-((u[2]^2+u[3]^2)*u[25]-(u[1]*u[2]-u[15])*u[26]-(u[1]*u[3]+u[14])*u[27])/g0
  anyib : Fcn  Expr=((u[1]*u[2]+u[15])*u[25]-(u[1]^2+u[3]^2)*u[26]+(u[2]*u[3]-u[13])*u[27])/g0
  anzib : Fcn  Expr=((u[1]*u[3]-u[14])*u[25]+(u[2]*u[3]+u[13])*u[26]-(u[1]^2+u[2]^2)*u[27])/g0
  mass cg inertia : Demux  Outputs=[1 3 4]
      settings: DisplayOption=none
  n : Fcn  Expr=-u[3]/(u[4]*g0)
  total : Demux  Outputs=[12 12]
      settings: DisplayOption=none
  xiacc : Constant  Value=xiacc
  yiacc : Constant  Value=yiacc
  ziacc : Constant  Value=ziacc
  yacc : Outport
  acc earth : Outport  Port=2
  wires:
  total/2 -> Terminator_13/1
  mass cg inertia/3 -> Terminator_12/1
  Demux2/4 -> Terminator_11/1
  Demux2/2 -> Terminator_10/1
  Demux1/2 -> Terminator_9/1
  Demux1/1 -> Terminator_8/1
  Demux/8 -> Terminator_7/1
  Demux/7 -> Terminator_6/1
  Demux/6 -> Terminator_5/1
  Demux/5 -> Terminator_4/1
  Demux/4 -> Terminator_3/1
  Demux/3 -> Terminator_2/1
  Demux/2 -> Terminator_1/1
  Mux4/1 -> yacc/1
  anb/1 -> Mux4/5
  Sum1/1 -> Mux1/3
  x/1 -> Mux1/1
  xdot/1 -> Mux1/2
  mass cg inertia/2 -> Sum1/1
  anzib/1 -> Mux3/3
  anxib/1 -> Mux3/1
  anyib/1 -> Mux3/2
  Mux2/1 -> n/1
  massinit/1 -> mass cg inertia/1
  xiacc/1 -> Mux/1
  yiacc/1 -> Mux/2
  ziacc/1 -> Mux/3
  1/(mg)/1 -> Prod1/2, Prod/2
  Sum/1 -> Prod1/1
  Mux1/1 -> anxib/1, anzib/1, anyib/1
  mass cg inertia/1 -> Mux2/2, 1/(mg)/1
  Mux/1 -> Sum1/2
  Mux3/1 -> Sum2/2
  Sum2/1 -> anib/1, Mux4/4
  FMa/1 -> Demux/1
  Fgr/1 -> Sum/2
  anib/1 -> Mux4/6
  n/1 -> Mux4/7
  total/1 -> Sum/1, Prod/1
  FMtot/1 -> total/1
  Demux/1 -> Mux2/1
  Demux2/3 -> Mux4/2, Sum2/1, anb/1
  Demux1/3 -> Mux4/1
  Prod/1 -> Demux1/1
  Demux2/1 -> Mux4/3
  Prod1/1 -> Demux2/1
  Demux1/4 -> acc earth/1

== system Citation_FlightGear_v2/Cessna Citation 500/Citation model DASMAT/AIRCRAFT MODEL/OBSERVATIONS/Energy ==
  x : Inport
  xdot : Inport  Port=2
  yatm : Inport  Port=3
  Mux : Mux  Inputs=[12 12 8]
  Mux1 : Mux  Inputs=2
  spec energy : Fcn  Expr=u[10]+(u[4]*u[4])/(2*u[28])
  spec power : Fcn  Expr=u[22]+(u[4]*u[16])/u[28]
  ys : Outport
  wires:
  spec power/1 -> Mux1/2
  spec energy/1 -> Mux1/1
  x/1 -> Mux/1
  xdot/1 -> Mux/2
  Mux1/1 -> ys/1
  yatm/1 -> Mux/3
  Mux/1 -> spec power/1, spec energy/1

== system Citation_FlightGear_v2/Cessna Citation 500/Citation model DASMAT/AIRCRAFT MODEL/OBSERVATIONS/Flight-Path ==
  x : Inport
  xdot : Inport  Port=2
  yuvw : Inport  Port=3
  acc earth : Inport  Port=4
  Demux : Demux  Outputs=[3 3 3 3]
      settings: DisplayOption=none
  Mux : Mux  Inputs=[12 12 3 3]
  Mux1 : Mux  Inputs=[30 1 1]
  Mux2 : Mux  Inputs=17
  Terminator11 : Terminator
  Terminator12 : Terminator
  Terminator13 : Terminator
  Vground : Fcn  Expr=sqrt(u[23]*u[23]+u[24]*u[24]+u[22]*u[22])
  bank angle : Fcn  Expr=asin(sin(u[7])*cos(u[8]))
  chi : Fcn  Expr=atan2(u[26],u[25])
  chidot : Fcn  Expr=(u[25]*u[29]*g0-u[28]*g0*u[26])/(u[4]*u[4]-u[27]*u[27])
  chimagn : Fcn  Expr=0
  chitrue : Fcn  Expr=atan2(u[24],u[23])
  chitruedot : Fcn  Expr=(u[23]*u[29]*g0-u[28]*g0*u[24])/(u[31]*u[31]-u[22]*u[22])
  flightpath acc : Fcn  Expr=u[16]/g0
  gamma : Fcn  Expr=asin(-u[27]/u[4])
  gammadot : Fcn  Expr=(-u[4]*u[30]*g0+u[16]*u[27])/(u[4]*sqrt(u[4]*u[4]-u[27]*u[27]))
  gammatrue : Fcn  Expr=asin(u[22]/u[31])
  gammatruedot : Fcn  Expr=(u[31]*u[32]*g0-u[16]*u[22])/(u[31]*sqrt(u[31]*u[31]-u[22]*u[22]))
  gsdev : Fcn  Expr=atan2(u[10]-hGS,sqrt((xGS-u[11])*(xGS-u[11])+(yGS-u[12])*(yGS-u[12]))) - 3*pi/180
  locdev : Fcn  Expr=psiLOC - atan2(yLOC-u[12],xLOC-u[11])
  psimagn : Fcn  Expr=0
  range : Fcn  Expr=sqrt((u[11]-xDME)*(u[11]-xDME)+(u[12]-yDME)*(u[12]-yDME)+(u[10]-hDME)*(u[10]-hDME))
  vertical acc : Fcn  Expr=-u[30]
  yfp : Outport
  wires:
  Demux/3 -> Terminator13/1
  Demux/2 -> Terminator12/1
  Demux/1 -> Terminator11/1
  vertical acc/1 -> Mux1/3, Mux2/16
  Mux1/1 -> gammatruedot/1, chitruedot/1, gammatrue/1, chitrue/1
  Vground/1 -> Mux1/2, Mux2/15
  xdot/1 -> Mux/2
  Demux/4 -> Mux/3
  acc earth/1 -> Mux/4
  yuvw/1 -> Demux/1
  chi/1 -> Mux2/2
  Mux2/1 -> yfp/1
  gamma/1 -> Mux2/1
  gammadot/1 -> Mux2/3
  chidot/1 -> Mux2/4
  gammatrue/1 -> Mux2/5
  chitrue/1 -> Mux2/6
  gammatruedot/1 -> Mux2/7
  flightpath acc/1 -> Mux2/17
  range/1 -> Mux2/14
  locdev/1 -> Mux2/13
  gsdev/1 -> Mux2/12
  bank angle/1 -> Mux2/11
  psimagn/1 -> Mux2/10
  chimagn/1 -> Mux2/9
  chitruedot/1 -> Mux2/8
  x/1 -> Mux/1
  Mux/1 -> Mux1/1, gammadot/1, chi/1, gamma/1, chidot/1, gsdev/1, locdev/1, range/1, Vground/1, vertical acc/1, flightpath acc/1, bank angle/1, psimagn/1, chimagn/1

== system Citation_FlightGear_v2/Cessna Citation 500/Citation model DASMAT/AIRCRAFT MODEL/WIND//TURBULENCE/Logarithmic Wind model ==
  In1 : Inport
  He Selector : Selector  InputPortWidth=12  IndexOptions=Index vector (dialog)  Indices=[10]  OutputSizes=1
  Logarithmic Wind model : Subsystem
  Mux : Mux  Inputs=3
  Out1 : Outport
  wires:
  In1/1 -> He Selector/1
  Mux/1 -> Out1/1
  Logarithmic Wind model/1(uwind) -> Mux/1  "uwind"
  Logarithmic Wind model/2(vwind) -> Mux/2  "vwind"
  Logarithmic Wind model/3(wwind) -> Mux/3  "wwind"
  He Selector/1 -> Logarithmic Wind model/1(he)

== system Citation_FlightGear_v2/Cessna Citation 500/Citation model DASMAT/AIRCRAFT MODEL/AFM/Aeromod/SubSystem ==
  x : Inport
  ua : Inport  Port=2
  cg : Inport  Port=3
  yad1 : Inport  Port=4
  yad2 : Inport  Port=5
  gust : Inport  Port=6
  yatm : Inport  Port=7
  0.30-dxcg/c : Fcn  Expr=0.3-(xcgref-u[1])/chord
  Ca : Demux  Outputs=6
      settings: DisplayOption=none
  Cadot : Demux  Outputs=6
      settings: DisplayOption=none
  Cag : Demux  Outputs=6
      settings: DisplayOption=none
  Cbdot : Demux  Outputs=6
      settings: DisplayOption=none
  Ground effect : Subsystem
  Saturation : Saturate  UpperLimit="[ 15  37  22  15  20  10 40 180/pi]*pi/180"  LowerLimit="[-20 -37 -22 -15 -20 -10 0  0]*pi/180"
  m/s2kts : Gain  Gain=[1 1 1 1 1 1.9438 1.9438 1.9438]  SaturateOnIntegerOverflow=on  OutDataTypeStr=Inherit: Same as input  ParamDataTypeStr=Inherit: Same as input
  model : Subsystem
  pqrnondims : Subsystem
  rud-rudtrim coupling : Subsystem
  CX : Outport
  CY : Outport  Port=2
  CZ : Outport  Port=3
  CLL : Outport  Port=4
  CM : Outport  Port=5
  CN : Outport  Port=6
  CXadot : Outport  Port=7
  CYadot : Outport  Port=8
  CZadot : Outport  Port=9
  CLLadot : Outport  Port=10
  CMadot : Outport  Port=11
  CNadot : Outport  Port=12
  CXbdot : Outport  Port=13
  CYbdot : Outport  Port=14
  CZbdot : Outport  Port=15
  CLLbdot : Outport  Port=16
  CMbdot : Outport  Port=17
  CNbdot : Outport  Port=18
  CXg : Outport  Port=19
  CYg : Outport  Port=20
  CZg : Outport  Port=21
  CLLg : Outport  Port=22
  CMg : Outport  Port=23
  CNg : Outport  Port=24
  wires:
  yad2/1 -> m/s2kts/1
  m/s2kts/1 -> model/7(yad2)
  Saturation/1 -> rud-rudtrim coupling/1(ua)
  model/4(Cag) -> Cag/1
  model/3(Cbdot) -> Cbdot/1
  Cbdot/2 -> CYbdot/1
  Cbdot/1 -> CXbdot/1
  Cbdot/3 -> CZbdot/1
  Cbdot/4 -> CLLbdot/1
  Cbdot/5 -> CMbdot/1
  Cbdot/6 -> CNbdot/1
  Cag/6 -> CNg/1
  Cag/5 -> CMg/1
  Cag/4 -> CLLg/1
  Cag/3 -> CZg/1
  Cag/1 -> CXg/1
  Cag/2 -> CYg/1
  model/2(Cadot) -> Cadot/1
  Cadot/2 -> CYadot/1
  Cadot/1 -> CXadot/1
  Cadot/3 -> CZadot/1
  Cadot/4 -> CLLadot/1
  Cadot/5 -> CMadot/1
  Cadot/6 -> CNadot/1
  Ca/6 -> CN/1
  Ca/5 -> CM/1
  Ca/4 -> CLL/1
  Ca/3 -> CZ/1
  Ca/1 -> CX/1
  Ca/2 -> CY/1
  model/1(Ca) -> Ca/1
  yad1/1 -> model/6(yad1)
  gust/1 -> model/8(gust)
  cg/1 -> 0.30-dxcg/c/1
  ua/1 -> Saturation/1
  x/1 -> pqrnondims/1(x), model/2(x)
  0.30-dxcg/c/1 -> model/5(dxcg/c)
  Ground effect/1(hcg) -> model/3(hcg)
  rud-rudtrim coupling/1(ua coupled) -> model/4(ua)
  pqrnondims/1(ypqrdl) -> model/1(ypqrdl)
  yatm/1 -> Ground effect/1(yatm)

== system Citation_FlightGear_v2/Cessna Citation 500/Citation model DASMAT/AIRCRAFT MODEL/AFM/FMaerodims/dims ==
  note: X,Y,Z
  FM/length : Inport
  Demux : Demux  Outputs=[12 3 3 3 3]
      settings: DisplayOption=none
  LL,M,N air : Gain  Gain=[span chord span]  SaturateOnIntegerOverflow=on  OutDataTypeStr=Inherit: Same as input  ParamDataTypeStr=Inherit: Same as input
  LL,M,N body : Gain  Gain=[span chord span]  SaturateOnIntegerOverflow=on  OutDataTypeStr=Inherit: Same as input  ParamDataTypeStr=Inherit: Same as input
  LL,M,N earth : Gain  Gain=[span chord span]  SaturateOnIntegerOverflow=on  OutDataTypeStr=Inherit: Same as input  ParamDataTypeStr=Inherit: Same as input
  LL,M,N stab : Gain  Gain=[span chord span]  SaturateOnIntegerOverflow=on  OutDataTypeStr=Inherit: Same as input  ParamDataTypeStr=Inherit: Same as input
  Mux : Mux  Inputs=[12 3 3 3 3]
  FM : Outport
  wires:
  LL,M,N earth/1 -> Mux/5
  Demux/5 -> LL,M,N earth/1
  LL,M,N body/1 -> Mux/4
  LL,M,N stab/1 -> Mux/3
  LL,M,N air/1 -> Mux/2
  Demux/1 -> Mux/1
  Demux/2 -> LL,M,N air/1
  Demux/3 -> LL,M,N stab/1
  Demux/4 -> LL,M,N body/1
  Mux/1 -> FM/1
  FM/length/1 -> Demux/1

== system Citation_FlightGear_v2/Cessna Citation 500/Citation model DASMAT/AIRCRAFT MODEL/AFM/FMaerodims/dims1 ==
  note: X,Y,Z
  F FM/length : Inport
  Demux : Demux  Outputs=[12 3 3 3 3]
      settings: DisplayOption=none
  LL,M,N air : Gain  Gain=[span chord span]  SaturateOnIntegerOverflow=on  OutDataTypeStr=Inherit: Same as input  ParamDataTypeStr=Inherit: Same as input
  LL,M,N body : Gain  Gain=[span chord span]  SaturateOnIntegerOverflow=on  OutDataTypeStr=Inherit: Same as input  ParamDataTypeStr=Inherit: Same as input
  LL,M,N earth : Gain  Gain=[span chord span]  SaturateOnIntegerOverflow=on  OutDataTypeStr=Inherit: Same as input  ParamDataTypeStr=Inherit: Same as input
  LL,M,N stab : Gain  Gain=[span chord span]  SaturateOnIntegerOverflow=on  OutDataTypeStr=Inherit: Same as input  ParamDataTypeStr=Inherit: Same as input
  Mux : Mux  Inputs=[12 3 3 3 3]
  FM : Outport
  wires:
  F FM/length/1 -> Demux/1
  Mux/1 -> FM/1
  Demux/4 -> LL,M,N body/1
  Demux/3 -> LL,M,N stab/1
  Demux/2 -> LL,M,N air/1
  Demux/1 -> Mux/1
  LL,M,N air/1 -> Mux/2
  LL,M,N stab/1 -> Mux/3
  LL,M,N body/1 -> Mux/4
  Demux/5 -> LL,M,N earth/1
  LL,M,N earth/1 -> Mux/5

== system Citation_FlightGear_v2/Cessna Citation 500/Citation model DASMAT/AIRCRAFT MODEL/AFM/FMaerodims/dims2 ==
  note: X,Y,Z
  F FM/length : Inport
  Demux : Demux  Outputs=[12 3 3 3 3]
      settings: DisplayOption=none
  LL,M,N air : Gain  Gain=[span chord span]  SaturateOnIntegerOverflow=on  OutDataTypeStr=Inherit: Same as input  ParamDataTypeStr=Inherit: Same as input
  LL,M,N body : Gain  Gain=[span chord span]  SaturateOnIntegerOverflow=on  OutDataTypeStr=Inherit: Same as input  ParamDataTypeStr=Inherit: Same as input
  LL,M,N earth : Gain  Gain=[span chord span]  SaturateOnIntegerOverflow=on  OutDataTypeStr=Inherit: Same as input  ParamDataTypeStr=Inherit: Same as input
  LL,M,N stab : Gain  Gain=[span chord span]  SaturateOnIntegerOverflow=on  OutDataTypeStr=Inherit: Same as input  ParamDataTypeStr=Inherit: Same as input
  Mux : Mux  Inputs=[12 3 3 3 3]
  FM : Outport
  wires:
  LL,M,N earth/1 -> Mux/5
  Demux/5 -> LL,M,N earth/1
  LL,M,N body/1 -> Mux/4
  LL,M,N stab/1 -> Mux/3
  LL,M,N air/1 -> Mux/2
  Demux/1 -> Mux/1
  Demux/2 -> LL,M,N air/1
  Demux/3 -> LL,M,N stab/1
  Demux/4 -> LL,M,N body/1
  Mux/1 -> FM/1
  F FM/length/1 -> Demux/1

== system Citation_FlightGear_v2/Cessna Citation 500/Citation model DASMAT/AIRCRAFT MODEL/AFM/FMgustdims/dims ==
  note: X,Y,Z
  F M/length : Inport
  Demux : Demux  Outputs=[12 3 3 3 3]
      settings: DisplayOption=none
  LL,M,N air : Gain  Gain=[span chord span]  SaturateOnIntegerOverflow=on  OutDataTypeStr=Inherit: Same as input  ParamDataTypeStr=Inherit: Same as input
  LL,M,N body : Gain  Gain=[span chord span]  SaturateOnIntegerOverflow=on  OutDataTypeStr=Inherit: Same as input  ParamDataTypeStr=Inherit: Same as input
  LL,M,N earth : Gain  Gain=[span chord span]  SaturateOnIntegerOverflow=on  OutDataTypeStr=Inherit: Same as input  ParamDataTypeStr=Inherit: Same as input
  LL,M,N stab : Gain  Gain=[span chord span]  SaturateOnIntegerOverflow=on  OutDataTypeStr=Inherit: Same as input  ParamDataTypeStr=Inherit: Same as input
  Mux : Mux  Inputs=[12 3 3 3 3]
  FM : Outport
  wires:
  LL,M,N earth/1 -> Mux/5
  Demux/5 -> LL,M,N earth/1
  LL,M,N body/1 -> Mux/4
  LL,M,N stab/1 -> Mux/3
  LL,M,N air/1 -> Mux/2
  Demux/1 -> Mux/1
  Demux/2 -> LL,M,N air/1
  Demux/3 -> LL,M,N stab/1
  Demux/4 -> LL,M,N body/1
  Mux/1 -> FM/1
  F M/length/1 -> Demux/1

== system Citation_FlightGear_v2/Cessna Citation 500/Citation model DASMAT/AIRCRAFT MODEL/EFM/Engmod/Citation eng_mod ==
  In1 : Inport
  Demux : Demux  Outputs=32
      settings: DisplayOption=none
  Mux : Mux  Inputs=6
  Mux1 : Mux  Inputs=2
  Subsystem1 : Subsystem
  Out1 : Outport
  ypp : Outport  Port=2
  wires:
  Subsystem1/4(MXt) -> Mux/4
  Subsystem1/3(Zt) -> Mux/3
  Subsystem1/2(Yt) -> Mux/2
  Subsystem1/1(Xt) -> Mux/1
  Subsystem1/6(MZt) -> Mux/6
  Subsystem1/5(MYt) -> Mux/5
  Mux/1 -> Out1/1
  In1/1 -> Demux/1
  Demux/1 -> Subsystem1/1(pbody)
  Demux/2 -> Subsystem1/2(qbody)
  Demux/3 -> Subsystem1/3(rbody)
  Demux/4 -> Subsystem1/4(VTAS)
  Demux/5 -> Subsystem1/5(alpha)
  Demux/6 -> Subsystem1/6(beta)
  Demux/7 -> Subsystem1/7(phi)
  Demux/8 -> Subsystem1/8(theta)
  Demux/9 -> Subsystem1/9(psi)
  Demux/10 -> Subsystem1/10(he)
  Demux/11 -> Subsystem1/11(xe)
  Demux/12 -> Subsystem1/12(ye)
  Demux/13 -> Subsystem1/13(ut1)
  Demux/14 -> Subsystem1/14(ut2)
  Demux/15 -> Subsystem1/15(pstat)
  Demux/16 -> Subsystem1/16(rho)
  Demux/17 -> Subsystem1/17(temp)
  Demux/18 -> Subsystem1/18(grav)
  Demux/19 -> Subsystem1/19(hpress)
  Demux/20 -> Subsystem1/20(hradio)
  Demux/21 -> Subsystem1/21(Hgeopot)
  Demux/22 -> Subsystem1/22(Vsound)
  Demux/23 -> Subsystem1/23(Mach)
  Demux/24 -> Subsystem1/24(qdyn)
  Demux/25 -> Subsystem1/25(Reynl)
  Demux/26 -> Subsystem1/26(qc)
  Demux/27 -> Subsystem1/27(qrel)
  Demux/28 -> Subsystem1/28(ptot)
  Demux/29 -> Subsystem1/29(temptot)
  Demux/30 -> Subsystem1/30(VEAS)
  Demux/31 -> Subsystem1/31(VCAS)
  Demux/32 -> Subsystem1/32(VIAS)
  Subsystem1/7(yppleft) -> Mux1/1
  Subsystem1/8(yppright) -> Mux1/2
  Mux1/1 -> ypp/1

== system Citation_FlightGear_v2/Cessna Citation 500/Citation model DASMAT/AIRCRAFT MODEL/EQM/State Derivatives/Vabdot ==
  x : Inport
  ypqr : Inport  Port=2
  Ftot : Inport  Port=3
  Fadot : Inport  Port=4
  Fbdot : Inport  Port=5
  mass : Inport  Port=6
  wind : Inport  Port=7
  Mux1 : Mux  Inputs=3
  Prod : Product  InputSameDT=on  SaturateOnIntegerOverflow=on  OutDataTypeStr=Inherit: Same as first input
  Prod1 : Product  InputSameDT=on  SaturateOnIntegerOverflow=on  OutDataTypeStr=Inherit: Same as first input
  Sum : Sum  Inputs=+++  InputSameDT=on  SaturateOnIntegerOverflow=on  OutDataTypeStr=Inherit: Same as first input
  Vdot : Subsystem
  abdot : Subsystem
  winddot : Derivative
  Vabdot : Outport
  Ftot corrected : Outport  Port=2
  wires:
  wind/1 -> winddot/1, Vdot/5(wind), abdot/7(wind)
  winddot/1 -> abdot/8(winddot), Vdot/6(winddot)
  Vdot/1(Vdot) -> Mux1/1
  mass/1 -> Vdot/4(mass), abdot/6(mass)
  ypqr/1 -> Vdot/2(ypqr), abdot/2(ypqr)
  x/1 -> Vdot/1(x), abdot/1(x)
  abdot/1(adot) -> Vdot/7(adot), Prod/2, Mux1/2
  abdot/2(bdot) -> Vdot/8(bdot), Prod1/2, Mux1/3
  Fbdot/1 -> abdot/5(Fbdot), Prod1/1
  Fadot/1 -> abdot/4(Fadot), Prod/1
  Prod1/1 -> Sum/3
  Mux1/1 -> Vabdot/1
  Sum/1 -> Vdot/3(Ftot), Ftot corrected/1
  Prod/1 -> Sum/2
  Ftot/1 -> abdot/3(Ftot), Sum/1

== system Citation_FlightGear_v2/Cessna Citation 500/Citation model DASMAT/AIRCRAFT MODEL/EQM/State Derivatives/eulerdot ==
  x : Inport
  Mux : Mux  Inputs=3
  phidot : Fcn  Expr=u[1]+tan(u[8])*(u[2]*sin(u[7])+u[3]*cos(u[7]))
  psidot : Fcn  Expr=(u[2]*sin(u[7])+u[3]*cos(u[7]))/cos(u[8])
  thetadot : Fcn  Expr=u[2]*cos(u[7])-u[3]*sin(u[7])
  eulerdot : Outport
  wires:
  x/1 -> phidot/1, psidot/1, thetadot/1
  Mux/1 -> eulerdot/1
  phidot/1 -> Mux/1
  thetadot/1 -> Mux/2
  psidot/1 -> Mux/3

== system Citation_FlightGear_v2/Cessna Citation 500/Citation model DASMAT/AIRCRAFT MODEL/EQM/State Derivatives/hxydot ==
  yuvw : Inport
  wind : Inport  Port=2
  Demux : Demux  Outputs=[3 3 3 3]
      settings: DisplayOption=none
  Demux1 : Demux  Outputs=[3 3 3 3]
      settings: DisplayOption=none
  Mux : Mux  Inputs=[3 3]
  Mux1 : Mux  Inputs=3
  Terminator_{1..6} (6 alike) : Terminator
  hedot : Fcn  Expr=-(u[3]+u[6])
  xedot : Fcn  Expr=u[1]+u[4]
  yedot : Fcn  Expr=u[2]+u[5]
  hxydot : Outport
  wires:
  Demux1/3 -> Terminator_6/1
  Demux1/2 -> Terminator_5/1
  Demux1/1 -> Terminator_4/1
  Demux/3 -> Terminator_3/1
  Demux/2 -> Terminator_2/1
  Demux/1 -> Terminator_1/1
  wind/1 -> Demux1/1
  Demux1/4 -> Mux/2
  yedot/1 -> Mux1/3
  xedot/1 -> Mux1/2
  hedot/1 -> Mux1/1  "hedot"
  Mux1/1 -> hxydot/1
  Mux/1 -> hedot/1, yedot/1, xedot/1
  yuvw/1 -> Demux/1
  Demux/4 -> Mux/1
